simulink model "lab6_sim"  (R2023b)
settings: Solver=VariableStepAuto  StartTime=0.0  StopTime=10  RelTol=1e-3
values from neighbouring files (symbols this model uses):
  denr = [1 r1 r0]    [lab4.m]
  J = 0.71*10^-3    (= 0.00071)    [lab4.m]
  ke = 0.33    [lab4.m]
  kEM = 0.01    [lab4.m]
  km = 0.33    [lab4.m]
  kp = 35    [lab4.m]
  La = 14.28*10^-3    (= 0.01428)    [lab4.m]
  nums = [s2 s1 s0]    [lab4.m]
  numt = [t2 0 0]    [lab4.m]
  Ra = 4.2    [lab4.m]
settings Model: Creator=ALEXANDRU  LastModifiedBy=ALEXANDRU

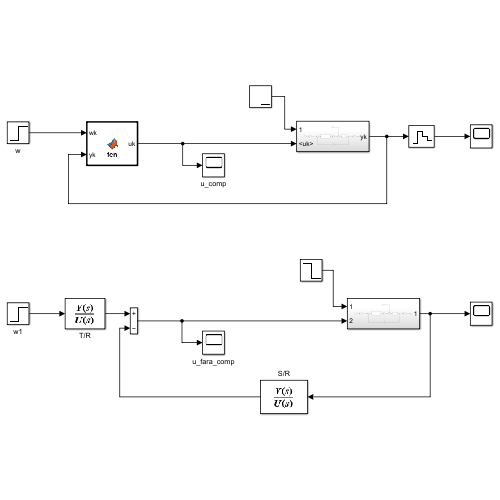
[thumbnail: Simulink's stored preview of the top-level diagram]
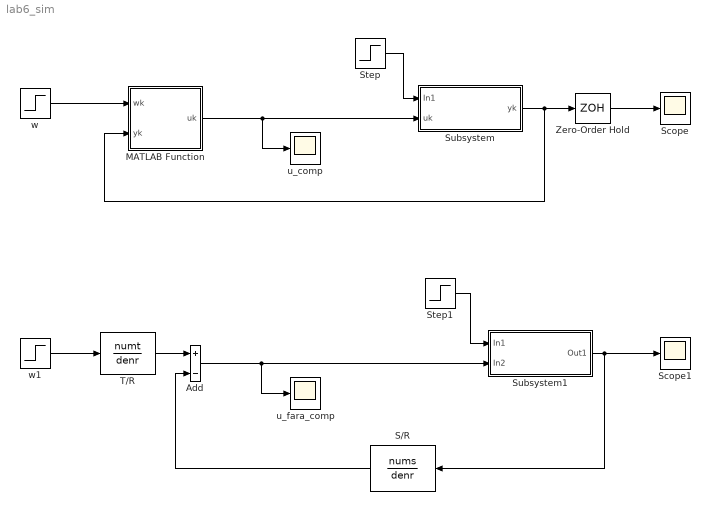
== system lab6_sim ==
  Add : Sum  Inputs=+-
  MATLAB Function : MATLAB Function  TreatAsAtomicUnit=on
  S/R : TransferFcn  Numerator=nums  Denominator=denr
  Scope : Scope
  Scope1 : Scope
  Step : Step  Time=0.6  After=-12  SampleTime=0
  Step1 : Step  Time=0.6  After=-12  SampleTime=0
  Subsystem : Subsystem
  Subsystem1 : Subsystem
  T/R : TransferFcn  Numerator=numt  Denominator=denr
  Zero-Order Hold : ZeroOrderHold  SampleTime=-1
  u_comp : Scope
  u_fara_comp : Scope
  w : Step  SampleTime=0
  w1 : Step  SampleTime=0
  wires:
  Step/1 -> Subsystem/1(In1)
  w/1 -> MATLAB Function/1(wk)
  Subsystem/1(yk) -> Zero-Order Hold/1, MATLAB Function/2(yk)
  MATLAB Function/1(uk) -> u_comp/1, Subsystem/2(uk)
  Zero-Order Hold/1 -> Scope/1
  w1/1 -> T/R/1
  Step1/1 -> Subsystem1/1(In1)
  Subsystem1/1(Out1) -> Scope1/1, S/R/1
  T/R/1 -> Add/1
  S/R/1 -> Add/2
  Add/1 -> Subsystem1/2(In2), u_fara_comp/1

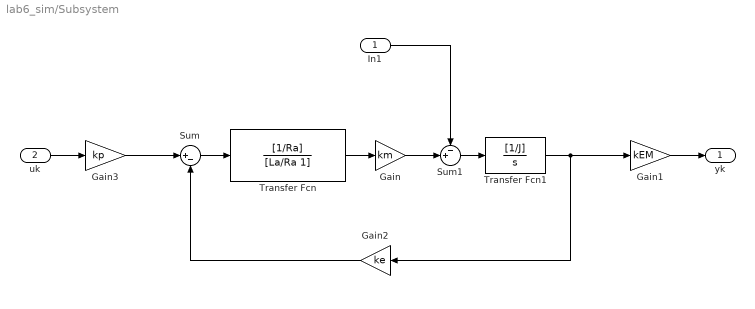
== system lab6_sim/Subsystem ==
  In1 : Inport
  uk : Inport  Port=2
  Gain : Gain  Gain=km
  Gain1 : Gain  Gain=kEM
  Gain2 : Gain  Gain=ke
  Gain3 : Gain  Gain=kp
  Sum : Sum  Inputs=|+-
  Sum1 : Sum  Inputs=-+|
  Transfer Fcn : TransferFcn  Numerator=[1/Ra]  Denominator=[La/Ra 1]
  Transfer Fcn1 : TransferFcn  Numerator=[1/J]  Denominator=[1 0]
  yk : Outport
  wires:
  Sum1/1 -> Transfer Fcn1/1
  Sum/1 -> Transfer Fcn/1
  Gain2/1 -> Sum/2
  Gain3/1 -> Sum/1
  Transfer Fcn/1 -> Gain/1
  Transfer Fcn1/1 -> Gain2/1, Gain1/1
  Gain/1 -> Sum1/2
  Gain1/1 -> yk/1
  In1/1 -> Sum1/1
  uk/1 -> Gain3/1

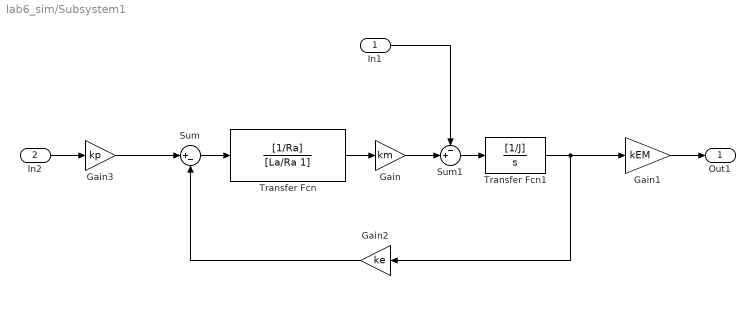
== system lab6_sim/Subsystem1 ==
  In1 : Inport
  In2 : Inport  Port=2
  Gain : Gain  Gain=km
  Gain1 : Gain  Gain=kEM
  Gain2 : Gain  Gain=ke
  Gain3 : Gain  Gain=kp
  Sum : Sum  Inputs=|+-
  Sum1 : Sum  Inputs=-+|
  Transfer Fcn : TransferFcn  Numerator=[1/Ra]  Denominator=[La/Ra 1]
  Transfer Fcn1 : TransferFcn  Numerator=[1/J]  Denominator=[1 0]
  Out1 : Outport
  wires:
  Sum1/1 -> Transfer Fcn1/1
  Sum/1 -> Transfer Fcn/1
  Gain2/1 -> Sum/2
  Gain3/1 -> Sum/1
  Transfer Fcn/1 -> Gain/1
  Transfer Fcn1/1 -> Gain2/1, Gain1/1
  Gain/1 -> Sum1/2
  Gain1/1 -> Out1/1
  In1/1 -> Sum1/1
  In2/1 -> Gain3/1

== matlab function lab6_sim/MATLAB Function ==
  settings: updateMethod=DISCRETE
  data: wk input; yk input; uk output; nums parameter; numt parameter; denr parameter
function uk = fcn(wk,yk,nums,numt,denr)
% nums = [s_2 s_1 s_0], numt = [t_2 0 0], denr = [1 r_1 r_0]

persistent ukm1 ukm2 ykm1 ykm2

if isempty(ukm1)
    % initializare variabile
    ukm1 = 0;
    ukm2 = 0;
    ykm1 = 0;
    ykm2 = 0;

end

uk = -denr(2)*ukm1-denr(3)*ukm2+numt(1)*wk-nums(1)*yk-nums(2)*ykm1-nums(3)*ykm2;

ukm2 = ukm1;
ukm1 = uk;
ukm2 = ykm1;
ykm1 = yk;

end
